simulink model "Herman_Problema2sim"  (R2021b)
settings: Solver=VariableStepAuto  StartTime=0.0  StopTime=70.0  RelTol=1e-3
values from neighbouring files (symbols this model uses):
  A = zeros(12)    [Herman_Problema2.m]
  Ad = expm(A*T)    [Herman_Problema2.m]
  B = zeros(12,4)    [Herman_Problema2.m]
  Bd = pinv(A) * (Ad - eye(12,12)) * B    [Herman_Problema2.m]
  C = zeros(6,12)    [Herman_Problema2.m]
  Cctrl = zeros(4,12)    [Herman_Problema2.m]
  Gd = pinv(A) * (Ad - eye(12,12)) * G    [Herman_Problema2.m]
  K = place(A,B,Pctrl)    [Herman_Problema2.m]
  k_bar = (Cctrl * (-A+B*K)^(-1)*B)^(-1)    [Herman_Problema2.m]
  phase = pi/2    (= 1.57079632679)    [Herman_Problema2.m]
  vk = 0.13    [Herman_Problema2.m]
  wk = [0.35;0.35;0.35;0.4;0.4;0.4]    [Herman_Problema2.m]
  x_bar = [0;0;0;0;2;0;0;0;0;0;0;0]    [Herman_Problema2.m]
  xh = [0;0;0;0;1.5;0;0;0;0;0;0;0]    [Herman_Problema2.m]
undefined symbols (not defined in the file or in its folder): DiscIntNeverNeededParam
libraries: simulink x1
settings Model: Creator=dr.gerardocastanon  LastModifiedBy=dr.gerardocastanon

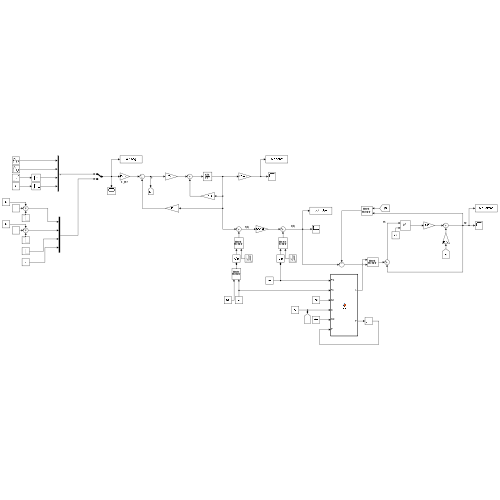
[thumbnail: Simulink's stored preview of the top-level diagram]
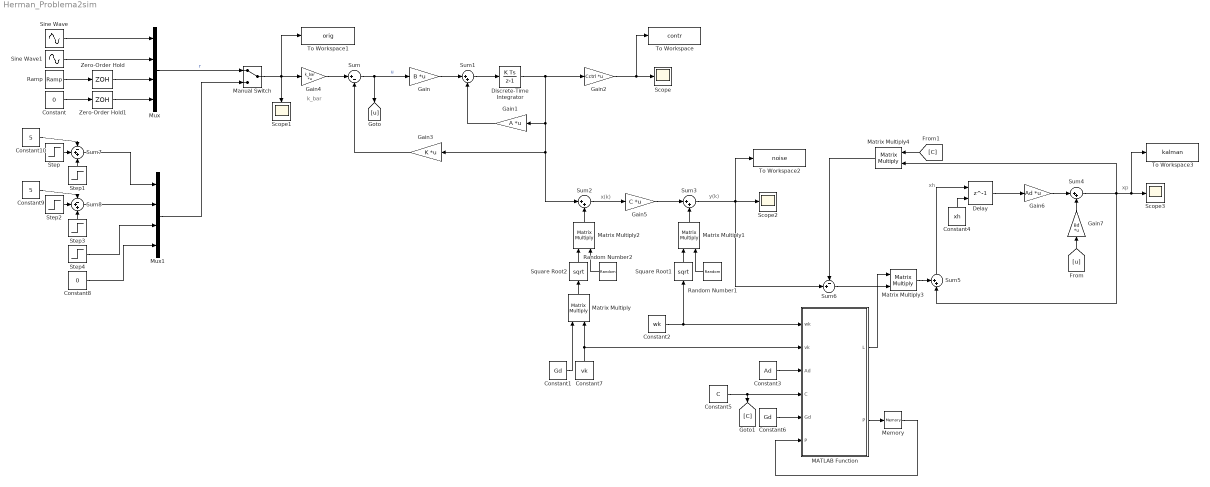
== system Herman_Problema2sim ==
  note: xp
  note: y(k)
  note: k_bar
  note: x(k)
  note: xh
  Constant : Constant  Value=0
  Constant1 : Constant  Value=Gd
  Constant10 : Constant  Value=5
  Constant2 : Constant  Value=wk
  Constant3 : Constant  Value=Ad
  Constant4 : Constant  Value=xh
  Constant5 : Constant  Value=C
  Constant6 : Constant  Value=Gd
  Constant7 : Constant  Value=vk
  Constant8 : Constant  Value=0  SampleTime=0.01
  Constant9 : Constant  Value=5
  Delay : Delay  DelayLength=1  InitialConditionSource=Input port  InitialCondition=xh  SampleTime=0.01
      settings: InputPortMap=u0,p4
  Discrete-Time Integrator : DiscreteIntegrator  InitialCondition=x_bar  SampleTime=-1  ICPrevOutput=DiscIntNeverNeededParam  ICPrevScaledInput=DiscIntNeverNeededParam
  Gain : Gain  Gain=B  Multiplication=Matrix(K*u)
  Gain1 : Gain  Gain=A  Multiplication=Matrix(K*u)
  Gain2 : Gain  Gain=Cctrl  Multiplication=Matrix(K*u) (u vector)
  Gain3 : Gain  Gain=K  Multiplication=Matrix(K*u) (u vector)
  Gain4 : Gain  Gain=k_bar  Multiplication=Matrix(K*u) (u vector)
  Gain5 : Gain  Gain=C  Multiplication=Matrix(K*u) (u vector)
  Gain6 : Gain  Gain=Ad  Multiplication=Matrix(K*u)
  Gain7 : Gain  Gain=Bd  Multiplication=Matrix(K*u)
  MATLAB Function : MATLAB Function  TreatAsAtomicUnit=on
  Manual Switch : ManualSwitch
  Matrix Multiply{,1..4} (5 alike) : Product  Multiplication=Matrix(*)
  Memory : Memory  InitialCondition=eye(12,12)
  Mux : Mux
  Mux1 : Mux
  Ramp : simulink/Sources/Ramp  slope=0.2  start=0  InitialOutput=0
  Random Number1 : RandomNumber  SampleTime=0.01
  Random Number2 : RandomNumber  SampleTime=0.01
  Scope{,1..3} (4 alike) : Scope
  Sine Wave : Sin  Amplitude=2  Frequency=0.2  Phase=phase  SampleTime=0.01
  Sine Wave1 : Sin  Amplitude=2  Frequency=0.2  SampleTime=0.01
  Square Root1 : Sqrt  SaturateOnIntegerOverflow=on
  Square Root2 : Sqrt  SaturateOnIntegerOverflow=on
  Step : Step  Time=10  After=5  SampleTime=0.01
  Step1 : Step  Time=30  Before=5  After=0  SampleTime=0.01
  Step2 : Step  Time=20  After=5  SampleTime=0.01
  Step3 : Step  Time=40  Before=5  After=0  SampleTime=0.01
  Step4 : Step  Time=50  Before=3  After=0  SampleTime=0.01
  Sum : Sum  Inputs=|+-
  Sum{1..4} (4 alike) : Sum  Inputs=|++
  Sum5 : Sum  Inputs=++|
  Sum6 : Sum  Inputs=-+|
  Sum7 : Sum  Inputs=-++
  Sum8 : Sum  Inputs=-++
  To Workspace : ToWorkspace  VariableName=contr  SampleTime=-1
  To Workspace1 : ToWorkspace  VariableName=orig  SampleTime=-1
  To Workspace2 : ToWorkspace  VariableName=noise  SampleTime=-1
  To Workspace3 : ToWorkspace  VariableName=kalman  SampleTime=-1
  Zero-Order Hold : ZeroOrderHold  SampleTime=0.01
  Zero-Order Hold1 : ZeroOrderHold  SampleTime=0.01
  wires:
  Sum/1 -> [u], Gain/1  "u"
  Gain3/1 -> Sum/2
  Gain4/1 -> Sum/1
  Gain2/1 -> To Workspace/1, Scope/1
  Gain/1 -> Sum1/1
  Gain1/1 -> Sum1/2
  Sine Wave/1 -> Mux/1
  Sine Wave1/1 -> Mux/2
  Sum1/1 -> Discrete-Time Integrator/1
  Discrete-Time Integrator/1 -> Gain1/1, Sum2/1, Gain3/1, Gain2/1
  Constant/1 -> Zero-Order Hold1/1
  Zero-Order Hold1/1 -> Mux/4
  Ramp/1 -> Zero-Order Hold/1
  Zero-Order Hold/1 -> Mux/3
  Sum2/1 -> Gain5/1
  Gain5/1 -> Sum3/1
  Sum3/1 -> Sum6/2, To Workspace2/1, Scope2/1
  Random Number1/1 -> Matrix Multiply1/2
  Square Root1/1 -> Matrix Multiply1/1
  Constant2/1 -> Square Root1/1, MATLAB Function/1(wk)
  Matrix Multiply1/1 -> Sum3/2
  Square Root2/1 -> Matrix Multiply2/1
  Matrix Multiply2/1 -> Sum2/2
  Random Number2/1 -> Matrix Multiply2/2
  Constant3/1 -> MATLAB Function/3(Ad)
  Constant5/1 -> MATLAB Function/4(C), [C]
  Constant6/1 -> MATLAB Function/5(Gd)
  Matrix Multiply/1 -> Square Root2/1
  Constant7/1 -> Matrix Multiply/2, MATLAB Function/2(vk)
  Constant1/1 -> Matrix Multiply/1
  MATLAB Function/2(P) -> Memory/1
  Memory/1 -> MATLAB Function/6("P ")
  Gain6/1 -> Sum4/1
  Gain7/1 -> Sum4/2
  Delay/1 -> Gain6/1
  [u] -> Gain7/1
  Sum4/1 -> Sum5/2, Matrix Multiply4/2, To Workspace3/1, Scope3/1
  Matrix Multiply4/1 -> Sum6/1
  [C] -> Matrix Multiply4/1
  Constant4/1 -> Delay/2
  Matrix Multiply3/1 -> Sum5/1
  Sum5/1 -> Delay/1
  MATLAB Function/1(L) -> Matrix Multiply3/1
  Sum6/1 -> Matrix Multiply3/2
  Constant10/1 -> Sum7/1
  Constant8/1 -> Mux1/4
  Step2/1 -> Sum8/2
  Step/1 -> Sum7/2
  Step3/1 -> Sum8/3
  Step1/1 -> Sum7/3
  Step4/1 -> Mux1/3
  Sum8/1 -> Mux1/2
  Constant9/1 -> Sum8/1
  Sum7/1 -> Mux1/1
  Mux1/1 -> Manual Switch/2
  Mux/1 -> Manual Switch/1  "r"
  Manual Switch/1 -> Gain4/1, Scope1/1, To Workspace1/1

== matlab function Herman_Problema2sim/MATLAB Function ==
  data: L output; P output; wk input; vk input; Ad input; C input; Gd input; P input
function [L,P] = fcn(wk,vk,Ad,C,Gd,P)

L = (Ad*P*Ad' + Gd*vk*Gd') * C' * pinv(C * (Ad*P*Ad' + Gd*vk*Gd') * C' + diag(wk));
P = (eye(12,12) - L*C) * (Ad*P*Ad' + Gd*diag(vk)*Gd') * (eye(12,12) - L*C)' + L*diag(wk)*L';
